simulink model "UR_template_effort"  (R2025a)
settings: Solver=VariableStepAuto  StartTime=0.0  StopTime=10  FixedStep=0.01  MaxStep=0.001  RelTol=1e-3
model workspace (MAT data in the model file):
  SL_ROS_VariableLengthArrays_MaxSizes : object (value not decoded)
undefined symbols (not defined in the file): data, data_SL_Info, T_desired_1, T_desired_2, T_desired_3
libraries: ros2lib x3
(part 2 of 2)

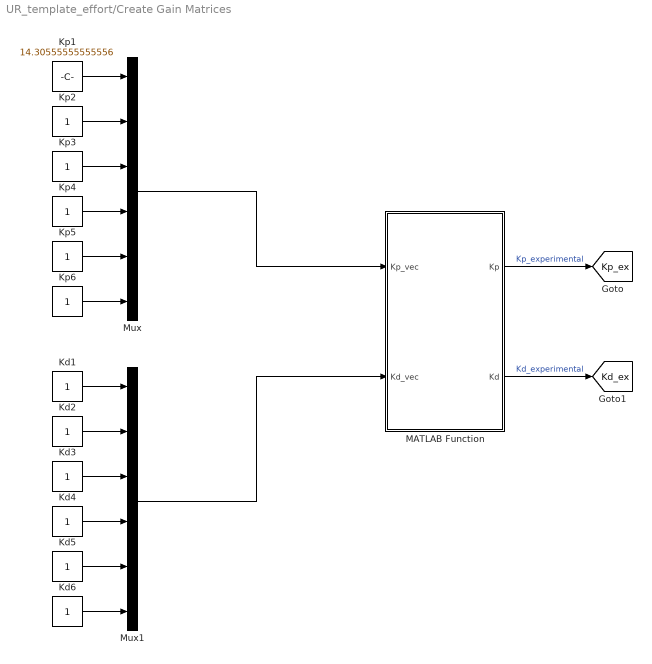
== system UR_template_effort/Create Gain Matrices ==
  Kd{1..6} (6 alike) : Constant
  Kp1 : Constant  Value=14.30555555555556
  Kp{2..6} (5 alike) : Constant
  MATLAB Function : MATLAB Function  TreatAsAtomicUnit=on
  Mux : Mux  Inputs=6
  Mux1 : Mux  Inputs=6
  tag scope: Kd_ex=global, Kp_ex=global
  wires:
  Kp5/1 -> Mux/5
  Kp6/1 -> Mux/6
  Kp4/1 -> Mux/4
  Kp3/1 -> Mux/3
  Kp2/1 -> Mux/2
  Kp1/1 -> Mux/1
  Mux/1 -> MATLAB Function/1(Kp_vec)
  Kd5/1 -> Mux1/5
  Kd1/1 -> Mux1/1
  Kd4/1 -> Mux1/4
  Kd3/1 -> Mux1/3
  Kd6/1 -> Mux1/6
  Kd2/1 -> Mux1/2
  Mux1/1 -> MATLAB Function/2(Kd_vec)
  MATLAB Function/1(Kp) -> [Kp_ex]  "Kp_experimental"
  MATLAB Function/2(Kd) -> [Kd_ex]  "Kd_experimental"

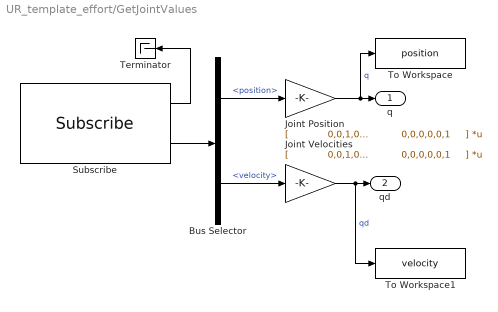
== system UR_template_effort/GetJointValues ==
  Bus Selector : BusSelector  OutputSignals=position,velocity
  Joint Position : Gain  Gain=|  Multiplication=Matrix(K*u) (u vector)
      | [
      |             0,0,1,0,0,0; 
      |             0,1,0,0,0,0; 
      |             1,0,0,0,0,0; 
      |             0,0,0,1,0,0; 
      |             0,0,0,0,1,0; 
      |             0,0,0,0,0,1
      |     ]
  Joint Velocities : Gain  Gain=|  Multiplication=Matrix(K*u) (u vector)
      | [
      |             0,0,1,0,0,0; 
      |             0,1,0,0,0,0; 
      |             1,0,0,0,0,0; 
      |             0,0,0,1,0,0; 
      |             0,0,0,0,1,0; 
      |             0,0,0,0,0,1
      |     ]
  Subscribe : ros2lib/Subscribe  topicSource=Select from ROS network  topic=/joint_states  messageType=sensor_msgs/JointState  sampleTime=-1  QOSHistory=Keep last  QOSDepth=10  QOSReliability=Reliable  QOSDurability=Volatile  QOSDeadline=Inf  QOSLifespan=Inf  QOSLiveliness=Automatic  QOSLeaseDuration=Inf  QOSAvoidROSNamespaceConventions=off
  Terminator : Terminator
  To Workspace : ToWorkspace  VariableName=position  SampleTime=-1
  To Workspace1 : ToWorkspace  VariableName=velocity  SampleTime=-1
  q : Outport
  qd : Outport  Port=2
  wires:
  Subscribe/2 -> Bus Selector/1
  Bus Selector/1 -> Joint Position/1  "<position>"
  Bus Selector/2 -> Joint Velocities/1  "<velocity>"
  Joint Position/1 -> To Workspace/1, q/1  "q"
  Subscribe/1 -> Terminator/1
  Joint Velocities/1 -> To Workspace1/1, qd/1  "qd"

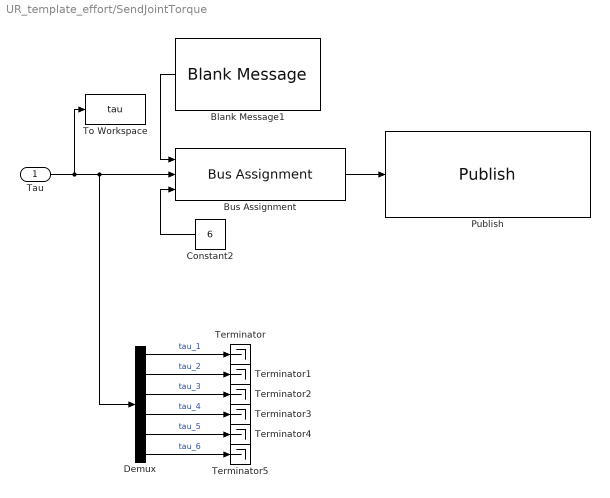
== system UR_template_effort/SendJointTorque ==
  Tau : Inport
  Blank Message1 : ros2lib/Blank Message  messageClass=Message  entityType=std_msgs/Float64MultiArray  messageType=std_msgs/Float64MultiArray  SampleTime=inf
  Bus Assignment : BusAssignment  AssignedSignals=data,data_SL_Info.CurrentLength
  Constant2 : Constant  Value=6  OutDataTypeStr=uint32
  Demux : Demux  Outputs=6
  Publish : ros2lib/Publish  topicSource=Select from ROS network  topic=/forward_effort_controller/commands  messageType=std_msgs/Float64MultiArray  QOSHistory=Keep last  QOSDepth=10  QOSReliability=Reliable  QOSDurability=Volatile  QOSDeadline=Inf  QOSLifespan=Inf  QOSLiveliness=Automatic  QOSLeaseDuration=Inf  QOSAvoidROSNamespaceConventions=off
  Terminator{,1..5} (6 alike) : Terminator
  To Workspace : ToWorkspace  VariableName=tau  SampleTime=-1
  wires:
  Constant2/1 -> Bus Assignment/3
  Blank Message1/1 -> Bus Assignment/1
  Bus Assignment/1 -> Publish/1
  Demux/2 -> Terminator1/1  "tau_2"
  Demux/3 -> Terminator2/1  "tau_3"
  Demux/1 -> Terminator/1  "tau_1"
  Tau/1 -> To Workspace/1, Demux/1, Bus Assignment/2
  Demux/5 -> Terminator4/1  "tau_5"
  Demux/6 -> Terminator5/1  "tau_6"
  Demux/4 -> Terminator3/1  "tau_4"

== matlab function UR_template_effort/Create Gain Matrices/MATLAB Function ==
  data: Kp_vec input; Kp output; Kd_vec input; Kd output
function [Kp,Kd] = fcn(Kp_vec, Kd_vec)
%#codegen

Kp = diag([Kp_vec]); 
Kd = diag([Kd_vec]); 
end
